simulink model "HvCoorn"  (R2022b)
settings: configuration reference "Icar05FusaMdlCfg" (kept outside this file)
undefined symbols (not defined in the file): BMSActSt_ACChrg, BMSActSt_DCChrg, BMSActSt_disconnect, BMSActSt_offline, BMSActSt_online, BMSActSt_undefined, BMSMainNegRlySt_Clsd_SC, BMSMainNegRlySt_Open_SC, BMSMainNegRlySt_StuckInClsd_SC, BMSMainNegRlySt_StuckInOpen_SC, BMSMainPosRlySt_Clsd_SC, BMSMainPosRlySt_Open_SC, BMSMainPosRlySt_StuckInClsd_SC, BMSPrecRlySt_StuckInOpen_SC, BMSReqSt_ACChrg, BMSReqSt_DCChrg, BMSReqSt_emergencyOffline, BMSReqSt_offline, BMSReqSt_online, Chrg_stCycleBookMod_SC, Chrg_stSingleBookMod_SC, CmpgMod_stInactv_SC, DCDCActSt_buck, DCDCActSt_connected, DCDCActSt_disconnected, DCDCReqSt_buck, DCDCReqSt_standby, EngStrtStop_RefuModDft_SC, EPBActSt_Appld_SC, GearLvr_stDrvGearD_SC, GearLvr_stDrvGearN_SC, GearLvr_stDrvGearP_SC, GearLvr_stDrvGearR_SC, hpp_bACChargeLinkIni_C, hpp_bACChargeLinkOKIni_C, hpp_bAcChgEnaIni_C, hpp_bAcChgPauseIni_C, hpp_bAcLinkTempErrIni_C, hpp_bBattWarmReqIni_C, hpp_bHvilHwErrIni_C, hpp_bHvilStOkIni_C, hpp_bHvRelayClsActIni_C, hpp_bHvRelayOpnActIni_C, hpp_bHvRelayStuckIni_C, hpp_bParked4ChDchgIni_C, hpp_bRemLvBatMntnReqIni_C, hpp_bStartUpReqIni_C, hpp_stHvilCanIni_C, hpp_stWarmTimeCfgRespIni_C, HvCoorn_bAuthEnaSwt_C, HvCoorn_bAuthFailSpdLimOvrd_C, HvCoorn_bAuthFailSpdLimOvrdVal_C, HvCoorn_bAuthStrt_C, HvCoorn_bBMSUnexpdDcnctFailEna_C, HvCoorn_bBuck2RdyBypDCDCEna_C, HvCoorn_bDCChrgFctCfg_C, HvCoorn_bDcChrgWkupEnaChrgLink_C, HvCoorn_bDCDcnct4ACEna_C, HvCoorn_bDCNotBuck2ShtdwnEna_C, HvCoorn_bDrvrLevNotRdyEna_C ... (+295)
libraries: ITKLib x213, simulink x61
(part 4 of 12)

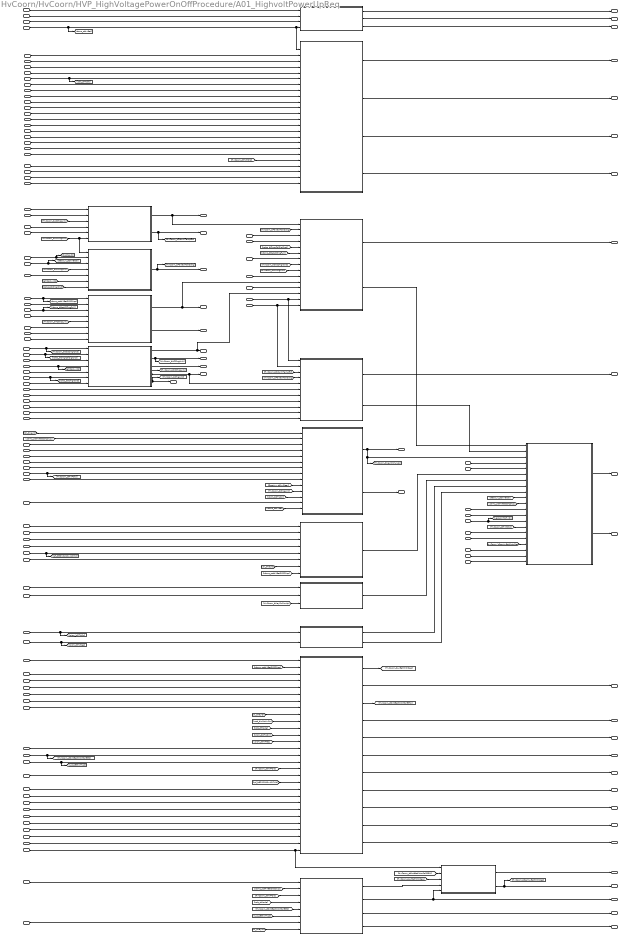
== system HvCoorn/HvCoorn/HVP_HighVoltagePowerOnOffProcedure/A01_HighvoltPowerUpReq ==
  HvCoorn_bHvReady : Inport
  BrkPedDev_bBrk : Inport  Port=2
  idi_bKeyOn : Inport  Port=3
  ian_tAcChrgrL1Temp : Inport  Port=4
  ian_tAcChrgrNTemp : Inport  Port=5
  icacu_stWarmTime : Inport  Port=6
  icbms_bBatACChrgFull : Inport  Port=7
  icbms_bStHvilSigErr : Inport  Port=8
  icbms_pctHVBatSOCDisp : Inport  Port=9
  icbms_stHvBat : Inport  Port=10
  icbms_stHvil : Inport  Port=11
  icbms_stMainNegRly : Inport  Port=12
  icbms_stMainPosRly : Inport  Port=13
  icbms_stPrecRly : Inport  Port=14
  icdc_bStHvilSigErr : Inport  Port=15
  icdc_stHvil : Inport  Port=16
  icdc_stMode : Inport  Port=17
  icfm_stMode : Inport  Port=18
  icobc_bChrgrCtrlSigCnct : Inport  Port=19
  icobc_bStAcHvilSigErr : Inport  Port=20
  icobc_pwrChrgMax : Inport  Port=21
  icobc_stHvil : Inport  Port=22
  HvCoorn_bObcChrgrCnct : Inport  Port=23
  icobc_stOBCMode : Inport  Port=24
  icobc_uChrgrCtrlSigVolt : Inport  Port=25
  icepb_stEpbSys : Inport  Port=26
  iczcu_stRmtChrgReq : Inport  Port=27
  Chrg_stBookChrgMod : Inport  Port=28
  ictel_stHvBatPrecdng : Inport  Port=29
  idi_bHvilInput : Inport  Port=30
  iud_bNoHVHWarmTiCfg : Inport  Port=31
  iud_bNoHVHConfig : Inport  Port=32
  iud_stOBCWakeUpOrigin : Inport  Port=33
  iud_stRemoteImmo : Inport  Port=34
  PwrLimBatt_pwrMaxHvesDChrg : Inport  Port=35
  Chrg_bACChrgCmpl : Inport  Port=36
  GearLvr_stDrvGear : Inport  Port=37
  VehSpd_vVeh : Inport  Port=38
  std_tExterTemp : Inport  Port=39
  HvCoorn_bHvilClsReqOld : Inport  Port=40
  tcj_bHvBatPrecdngFinish : Inport  Port=41
  inv_stHvBattWarmTime : Inport  Port=42
  icbms_stDcChrgrCnct : Inport  Port=43
  ian_tDcChrgrTemp1 : Inport  Port=44
  ian_tDcChrgrTemp2 : Inport  Port=45
  Chrg_bDCChrgCmpl : Inport  Port=46
  icbms_bBatDCChrgFull : Inport  Port=47
  icbms_uDcChgrCap : Inport  Port=48
  icbms_iDcChgrCap : Inport  Port=49
  icbms_bDcChrgCfg : Inport  Port=50
  icrm_stMode : Inport  Port=51
  VehCfg_bFrntMotByp : Inport  Port=52
  idi_bKeyStrt : Inport  Port=53
  icbms_bDcChrgWkup : Inport  Port=54
  Chrg_bChrgErrForever : Inport  Port=55
  icbms_bHvShutOffReq : Inport  Port=56
  iczcu_bHVPwrOffReq : Inport  Port=57
  icecc_bHVReq : Inport  Port=58
  HvCoorn_stHVPOld : Inport  Port=59
  icecc_bWPTCHvilFlt : Inport  Port=60
  icecc_bEASHvilFlt : Inport  Port=61
  icicm_bPwrOffReq : Inport  Port=62
  ved_bHvShtdwn : Inport  Port=63
  ipf_bBD1CAN0x41CVld : Inport  Port=64
  icicm_bOTAOn : Inport  Port=65
  icicm_stHVReq : Inport  Port=66
  icobc_bDchrgrCnct : Inport  Port=67
  ictcp_stRmtHvReq : Inport  Port=68
  iczcu_stCarMod : Inport  Port=69
  HvCoorn_bV2LActv : Inport  Port=70
  HvCoorn_bHvInitFail : Inport  Port=71
  HvCoorn_bHvOnFai : Inport  Port=72
  ved_bInhbHvOn : Inport  Port=73
  Chrg_bChrgStopBySOCLim : Inport  Port=74
  Chrg_bBookChrgCmpl : Inport  Port=75
  icobc_bVehCnct : Inport  Port=76
  icfm_bHvilFlt : Inport  Port=77
  icrm_bHvilFlt : Inport  Port=78
  icebs_pctLvBatSoh : Inport  Port=79
  icbms_tMaxBat : Inport  Port=80
  icbms_tMinBat : Inport  Port=81
  icebs_tLvBat : Inport  Port=82
  icebs_pctLvBatSoc : Inport  Port=83
  icebs_stSocPrcsn : Inport  Port=84
  icebs_uLvBat : Inport  Port=85
  icicm_stOTAPwrMngtReq : Inport  Port=86
  HvCoorn_ctSmtBatMntnFailEER : Inport  Port=87
  iud_bEEIniFnsd : Inport  Port=88
  HvCoorn_ctSmtBatMntnSucsEER : Inport  Port=89
  iclbms_stLvRemChrgReq : Inport  Port=90
  ipf_bLBMSCANVld : Inport  Port=91
  VehCfg_stLvBattTyp : Inport  Port=92
  icisg_bHvilFlt : Inport  Port=93
  idi_uPwrSply : Inport  Port=94
  ipf_bLIN9EBS0x34NodLostErr : Inport  Port=95
  HvCoorn_bSocWkupEER : Inport  Port=96
  HvCoorn_bTimerWkupReqEER : Inport  Port=97
  HvCoorn_stRemLvBatMntnFailRsnEER : Inport  Port=98
  icems_bFanAftRunActv : Inport  Port=99
  RngPrdn_volFuRmnByInstModEEW : Inport  Port=100
  ved_bInhbEngStrt : Inport  Port=101
  idi_bEBSLinWkup : Inport  Port=102
  idi_bTimerWkup : Inport  Port=103
  HvCoorn_pctHVBatSocEER : Inport  Port=104
  idi_noBMSSocCounter : Inport  Port=105
  DrvMod_bVehShowMod : Inport  Port=106
  icisg_uAct : Inport  Port=107
  icrm_uAct : Inport  Port=108
  icecc_uPTCAct : Inport  Port=109
  icecc_uEASAct : Inport  Port=110
  ved_bCellVoltUndLimSrus : Inport  Port=111
  B01_HvRelayClsAct : Subsystem  Description=高压继电器状态确认
  B02_HvilStCal : Subsystem  Description=互锁状态确认
  B03_ChgrPortOverTemp : Subsystem  Description=充电连接温度故障
  B04_ParkCheck : Subsystem  Description=停车检测
  B05_BattWarmReq : Subsystem
  B06_ChgrCnctStCal : Subsystem  Description=充电连接状态确认
  B07_AcChrgPwrUp : Subsystem  Description=AC充电上高压
  B08_DcChrgPwrUp : Subsystem  Description=DC充电上高压
  B09_KeyOnPwrUp : Subsystem  Description=KeyOn上高压
  B10_RemotePwrUp : Subsystem
  B11_ECCPwrUp : Subsystem  Description=热管理上高压
  B12_OTAPwrUp : Subsystem
  B13_GatherPwrUpReq : Subsystem  Description=高压上电请求
  B14_SmtLvBatMntn : Subsystem
  B15_LbmsMntn : Subsystem
  B16_LvBattTypSwt : Subsystem
  HvCoorn_bACChrgLink : Outport  VectorParamsAs1DForOutWhenUnconnected=off
  HvCoorn_bACChrgLinkOk : Outport  Port=2  VectorParamsAs1DForOutWhenUnconnected=off
  HvCoorn_stHvil : Outport  Port=3  VectorParamsAs1DForOutWhenUnconnected=off
  HvCoorn_bHvilHwStOk : Outport  Port=4  VectorParamsAs1DForOutWhenUnconnected=off
  HvCoorn_bHvilStOk : Outport  Port=5  VectorParamsAs1DForOutWhenUnconnected=off
  HvCoorn_bACChrgPause : Outport  Port=6  VectorParamsAs1DForOutWhenUnconnected=off
  HvCoorn_bHvRlyClsAct : Outport  Port=7  VectorParamsAs1DForOutWhenUnconnected=off
  HvCoorn_bHvRlyOpenAct : Outport  Port=8  VectorParamsAs1DForOutWhenUnconnected=off
  HvCoorn_bHvRlyStuck : Outport  Port=9  VectorParamsAs1DForOutWhenUnconnected=off
  HvCoorn_bACLinkTempErr : Outport  Port=10  VectorParamsAs1DForOutWhenUnconnected=off
  HvCoorn_bParked4ChDchg : Outport  Port=11  VectorParamsAs1DForOutWhenUnconnected=off
  HvCoorn_bBattWarmReq : Outport  Port=12  VectorParamsAs1DForOutWhenUnconnected=off
  HvCoorn_stWarmTimeCfgResp : Outport  Port=13  VectorParamsAs1DForOutWhenUnconnected=off
  HvCoorn_bACChrgEna : Outport  Port=14  VectorParamsAs1DForOutWhenUnconnected=off
  HvCoorn_bRemLvBatMntnReq : Outport  Port=15  VectorParamsAs1DForOutWhenUnconnected=off
  HvCoorn_bDCChrgLink : Outport  Port=16  VectorParamsAs1DForOutWhenUnconnected=off
  HvCoorn_bChrgLink : Outport  Port=17  VectorParamsAs1DForOutWhenUnconnected=off
  HvCoorn_bDCLinkTempErr : Outport  Port=18  VectorParamsAs1DForOutWhenUnconnected=off
  HvCoorn_bDCChrgEna : Outport  Port=19  VectorParamsAs1DForOutWhenUnconnected=off
  HvCoorn_stStartUpReq : Outport  Port=20  VectorParamsAs1DForOutWhenUnconnected=off
  HvCoorn_bCtrlrHvilErr : Outport  Port=21  VectorParamsAs1DForOutWhenUnconnected=off
  HvCoorn_bKeyOnPwrUp : Outport  Port=22  VectorParamsAs1DForOutWhenUnconnected=off
  HvCoorn_bSocWkup : Outport  Port=23  VectorParamsAs1DForOutWhenUnconnected=off
  HvCoorn_ctSmtBatMntnFailEEW : Outport  Port=24  VectorParamsAs1DForOutWhenUnconnected=off
  HvCoorn_stRemLvBatMntnFailRsn : Outport  Port=25  VectorParamsAs1DForOutWhenUnconnected=off
  HvCoorn_ctSmtBatMntnSucsEEW : Outport  Port=26  VectorParamsAs1DForOutWhenUnconnected=off
  HvCoorn_bTimerWkupReq : Outport  Port=27  VectorParamsAs1DForOutWhenUnconnected=off
  HvCoorn_bLbmsLvBatMntnReq : Outport  Port=28  VectorParamsAs1DForOutWhenUnconnected=off
  HvCoorn_pctLbmsSocMntnThd : Outport  Port=29  VectorParamsAs1DForOutWhenUnconnected=off
  HvCoorn_bLbmsSocWkup : Outport  Port=30  VectorParamsAs1DForOutWhenUnconnected=off
  HvCoorn_bVehNetWkupEna : Outport  Port=31  VectorParamsAs1DForOutWhenUnconnected=off
  HvCoorn_bSocWkupEEW : Outport  Port=32  VectorParamsAs1DForOutWhenUnconnected=off
  HvCoorn_bTimerWkupReqEEW : Outport  Port=33  VectorParamsAs1DForOutWhenUnconnected=off
  HvCoorn_stRemLvBatMntnFailRsnEEW : Outport  Port=34  VectorParamsAs1DForOutWhenUnconnected=off
  HvCoorn_pctHVBatSocEEW : Outport  Port=35  VectorParamsAs1DForOutWhenUnconnected=off
  HvCoorn_bShowModSocLo : Outport  Port=36  VectorParamsAs1DForOutWhenUnconnected=off
  HvCoorn_bStartUpReq : Outport  Port=37  VectorParamsAs1DForOutWhenUnconnected=off
  wires:
  B06_ChgrCnctStCal/2(HvCoorn_bACChrgLink) -> [HvCoorn_bACChrgLink], HvCoorn_bACChrgLink/1
  icdc_bStHvilSigErr/1 -> B02_HvilStCal/3(icdc_bStHvilSigErr)
  icobc_bStAcHvilSigErr/1 -> B02_HvilStCal/4(icobc_bStAcHvilSigErr)
  icbms_bStHvilSigErr/1 -> B02_HvilStCal/2(icbms_bStHvilSigErr)
  icdc_stMode/1 -> [icdc_stMode], B02_HvilStCal/6(icdc_stMode)
  icobc_stOBCMode/1 -> B02_HvilStCal/7(icobc_stOBCMode)
  idi_bHvilInput/1 -> B02_HvilStCal/8(idi_bHvilInput)
  icbms_stHvil/1 -> B02_HvilStCal/9(icbms_stHvil)
  icdc_stHvil/1 -> B02_HvilStCal/10(icdc_stHvil)
  icobc_stHvil/1 -> B02_HvilStCal/11(icobc_stHvil)
  B02_HvilStCal/3(HvCoorn_stHvil) -> HvCoorn_stHvil/1
  B02_HvilStCal/2(HvCoorn_bHvilHwStOk) -> HvCoorn_bHvilHwStOk/1
  B02_HvilStCal/1(HvCoorn_bHvilStOk) -> HvCoorn_bHvilStOk/1
  HvCoorn_bObcChrgrCnct/1 -> B06_ChgrCnctStCal/1(HvCoorn_bObcChrgrCnct), [HvCoorn_bObcChrgrCnct]
  icobc_bChrgrCtrlSigCnct/1 -> B06_ChgrCnctStCal/2(icobc_bChrgrCtrlSigCnct), [icobc_bChrgrCtrlSigCnct]
  VehSpd_vVeh/1 -> [VehSpd_vVeh], B06_ChgrCnctStCal/4(VehSpd_vVeh)
  icobc_uChrgrCtrlSigVolt/1 -> B06_ChgrCnctStCal/3(icobc_uChrgrCtrlSigVolt)
  B06_ChgrCnctStCal/3(HvCoorn_bACChrgPause) -> HvCoorn_bACChrgPause/1
  icfm_stMode/1 -> B02_HvilStCal/5(icfm_stMode)
  icbms_stHvBat/1 -> [icbms_stHvBat], B02_HvilStCal/1(icbms_stHvBat), B01_HvRelayClsAct/4(icbms_stHvBat)
  icbms_stMainPosRly/1 -> B01_HvRelayClsAct/1(icbms_stMainPosRly)
  icbms_stPrecRly/1 -> B01_HvRelayClsAct/2(icbms_stPrecRly)
  icbms_stMainNegRly/1 -> B01_HvRelayClsAct/3(icbms_stMainNegRly)
  B01_HvRelayClsAct/1(HvCoorn_bHvRlyClsAct) -> HvCoorn_bHvRlyClsAct/1
  B01_HvRelayClsAct/2(HvCoorn_bHvRlyOpenAct) -> HvCoorn_bHvRlyOpenAct/1
  B01_HvRelayClsAct/3(HvCoorn_bHvRlyStuck) -> HvCoorn_bHvRlyStuck/1
  ian_tAcChrgrL1Temp/1 -> B03_ChgrPortOverTemp/1(ian_tAcChrgrL1Temp)
  ian_tAcChrgrNTemp/1 -> B03_ChgrPortOverTemp/2(ian_tAcChrgrNTemp)
  [HvCoorn_bACChrgLink] -> B03_ChgrPortOverTemp/3(HvCoorn_bACChrgLink)
  [HvCoorn_bACChrgLink] -> B04_ParkCheck/4(HvCoorn_bACChrgLink)
  icepb_stEpbSys/1 -> B04_ParkCheck/5(icepb_stEpbSys)
  GearLvr_stDrvGear/1 -> B04_ParkCheck/3(GearLvr_stDrvGear), [GearLvr_stDrvGear]
  idi_bKeyOn/1 -> B04_ParkCheck/2(idi_bKeyOn), [idi_bKeyOn]
  Chrg_stBookChrgMod/1 -> B07_AcChrgPwrUp/7(Chrg_stBookChrgMod)
  B05_BattWarmReq/1(HvCoorn_bBattWarmReq) -> HvCoorn_bBattWarmReq/1, B07_AcChrgPwrUp/11(HvCoorn_bBattWarmReq)
  std_tExterTemp/1 -> B05_BattWarmReq/2(std_tExterTemp)
  [HvCoorn_bACChrgLink] -> B05_BattWarmReq/5(HvCoorn_bACChrgLink)
  icbms_bBatACChrgFull/1 -> [icbms_bBatACChrgFull], B05_BattWarmReq/3(icbms_bBatACChrgFull)
  B05_BattWarmReq/2(HvCoorn_stWarmTimeCfgResp) -> HvCoorn_stWarmTimeCfgResp/1
  icacu_stWarmTime/1 -> B05_BattWarmReq/4(icacu_stWarmTime)
  icbms_pctHVBatSOCDisp/1 -> B05_BattWarmReq/1(icbms_pctHVBatSOCDisp), [icbms_pctHVBatSOCDisp]
  B07_AcChrgPwrUp/1(HvCoorn_bACChrgEna) -> HvCoorn_bACChrgEna/1
  B03_ChgrPortOverTemp/1(HvCoorn_bACLinkTempErr) -> HvCoorn_bACLinkTempErr/1, B07_AcChrgPwrUp/1(HvCoorn_bACLinkTempErr)
  HvCoorn_bHvilClsReqOld/1 -> B02_HvilStCal/12(HvCoorn_bHvilClsReq)
  iud_bNoHVHConfig/1 -> B05_BattWarmReq/6(iud_bNoHVHConfig)
  iud_bNoHVHWarmTiCfg/1 -> B05_BattWarmReq/7(iud_bNoHVHWarmTiCfg)
  inv_stHvBattWarmTime/1 -> B05_BattWarmReq/8(inv_stHvBattWarmTime)
  PwrLimBatt_pwrMaxHvesDChrg/1 -> B09_KeyOnPwrUp/3(PwrLimBatt_pwrMaxHvesDChrg)
  [icbms_pctHVBatSOCDisp] -> B09_KeyOnPwrUp/2(icbms_pctHVBatSOCDisp)
  iud_stRemoteImmo/1 -> B10_RemotePwrUp/4(iud_stRemoteImmo)
  iczcu_stRmtChrgReq/1 -> B10_RemotePwrUp/3(iczcu_stRmtChrgReq)
  tcj_bHvBatPrecdngFinish/1 -> B10_RemotePwrUp/2(tcj_bHvBatPrecdngFinish)
  ictel_stHvBatPrecdng/1 -> B10_RemotePwrUp/1(ictel_stHvBatPrecdng)
  B10_RemotePwrUp/1(HvCoorn_bRemPwrUp) -> B13_GatherPwrUpReq/6(HvCoorn_bRemPwrUp)
  B09_KeyOnPwrUp/1(HvCoorn_bKeyOnPwrUp) -> [HvCoorn_bKeyOnPwrUp], B13_GatherPwrUpReq/3(HvCoorn_bKeyOnPwrUp), HvCoorn_bKeyOnPwrUp/1
  B07_AcChrgPwrUp/2(HvCoorn_bACChrgPwrUp) -> B13_GatherPwrUpReq/1(HvCoorn_bACChrgPwrUp)
  [idi_bKeyOn] -> B09_KeyOnPwrUp/1(idi_bKeyOn)
  icobc_pwrChrgMax/1 -> B07_AcChrgPwrUp/10(icobc_pwrChrgMax)
  [HvCoorn_bObcChrgrCnct] -> B07_AcChrgPwrUp/8(HvCoorn_bObcChrgrCnct)
  [icbms_bBatACChrgFull] -> B07_AcChrgPwrUp/6(icbms_bBatACChrgFull)
  [icobc_bChrgrCtrlSigCnct] -> B07_AcChrgPwrUp/5(icobc_bChrgrCtrlSigCnct)
  iud_stOBCWakeUpOrigin/1 -> B07_AcChrgPwrUp/4(iud_stOBCWakeUpOrigin)
  Chrg_bACChrgCmpl/1 -> B07_AcChrgPwrUp/3(Chrg_bACChrgCmpl)
  [HvCoorn_bACChrgLink] -> B07_AcChrgPwrUp/9(HvCoorn_bACChrgLink)
  B06_ChgrCnctStCal/1(HvCoorn_bACChrgLinkOk) -> HvCoorn_bACChrgLinkOk/1, B07_AcChrgPwrUp/13(HvCoorn_bACChrgLinkOk)
  icbms_stDcChrgrCnct/1 -> B06_ChgrCnctStCal/5(icbms_stDcChrgrCnct)
  B06_ChgrCnctStCal/4(HvCoorn_bDCChrgLink) -> [HvCoorn_bDCChrgLink], HvCoorn_bDCChrgLink/1, B08_DcChrgPwrUp/5(HvCoorn_bDCChrgLink)
  B06_ChgrCnctStCal/5(HvCoorn_bChrgLink) -> [HvCoorn_bChrgLink], HvCoorn_bChrgLink/1
  B08_DcChrgPwrUp/2(HvCoorn_bDCChrgPwrUp) -> B13_GatherPwrUpReq/2(HvCoorn_bDCChrgPwrUp)
  [HvCoorn_bDCChrgLink] -> B04_ParkCheck/1(HvCoorn_bDCChrgLink), B03_ChgrPortOverTemp/6(HvCoorn_bDCChargeLink)
  ian_tDcChrgrTemp1/1 -> B03_ChgrPortOverTemp/4(ian_tDcChrgrTemp1)
  ian_tDcChrgrTemp2/1 -> B03_ChgrPortOverTemp/5(ian_tDcChrgrTemp2)
  B03_ChgrPortOverTemp/2(HvCoorn_bDCLinkTempErr) -> [HvCoorn_bDcLinkTempErr], HvCoorn_bDCLinkTempErr/1
  [HvCoorn_bDcLinkTempErr] -> B08_DcChrgPwrUp/3(HvCoorn_bDcLinkTempErr)
  [HvCoorn_bParked4ChDchg] -> B08_DcChrgPwrUp/4(HvCoorn_bParked4ChDchg)
  B04_ParkCheck/1(HvCoorn_bParked4ChDchg) -> HvCoorn_bParked4ChDchg/1, [HvCoorn_bParked4ChDchg]
  icbms_bDcChrgCfg/1 -> B08_DcChrgPwrUp/6(icbms_bDcChrgCfg)
  Chrg_bDCChrgCmpl/1 -> B08_DcChrgPwrUp/7(Chrg_bDCChrgCmpl)
  icbms_bBatDCChrgFull/1 -> B08_DcChrgPwrUp/8(icbms_bBatDCChrgFull)
  icbms_uDcChgrCap/1 -> B08_DcChrgPwrUp/9(icbms_uDcChgrCap)
  icbms_iDcChgrCap/1 -> B08_DcChrgPwrUp/10(icbms_iDcChgrCap)
  B08_DcChrgPwrUp/1(HvCoorn_bDCChrgEna) -> HvCoorn_bDCChrgEna/1
  [HvCoorn_bParked4ChDchg] -> B07_AcChrgPwrUp/2(HvCoorn_bParked4ChDchg)
  icrm_stMode/1 -> B02_HvilStCal/13(icrm_stMode)
  VehCfg_bFrntMotByp/1 -> B02_HvilStCal/14(VehCfg_bFrntMotByp)
  idi_bKeyStrt/1 -> B09_KeyOnPwrUp/4(idi_bKeyStrt)
  icbms_bDcChrgWkup/1 -> B08_DcChrgPwrUp/11(icbms_bDcChrgWkup)
  HvCoorn_bHvReady/1 -> B09_KeyOnPwrUp/5(HvCoorn_bHvReady)
  BrkPedDev_bBrk/1 -> B09_KeyOnPwrUp/6(BrkPedDev_bBrk)
  [VehSpd_vVeh] -> B04_ParkCheck/6(VehSpd_vVeh)
  Chrg_bChrgErrForever/1 -> B08_DcChrgPwrUp/2(Chrg_bChrgErrForever), B07_AcChrgPwrUp/15(Chrg_bChrgErrForever)
  icbms_bHvShutOffReq/1 -> B13_GatherPwrUpReq/5(icbms_bHvShutOffReq)
  iczcu_bHVPwrOffReq/1 -> B09_KeyOnPwrUp/7(iczcu_bHVPwrOffReq)
  icecc_bHVReq/1 -> B11_ECCPwrUp/1(icecc_bHVReq)
  B11_ECCPwrUp/1(HvCoorn_bECCPwrUp) -> B13_GatherPwrUpReq/7(HvCoorn_bECCPwrUp)
  B13_GatherPwrUpReq/1(HvCoorn_bStartUpReq) -> HvCoorn_bStartUpReq/1
  HvCoorn_stHVPOld/1 -> [HvCoorn_stHVPOld], B09_KeyOnPwrUp/8(HvCoorn_stHVPOld)
  icecc_bWPTCHvilFlt/1 -> B02_HvilStCal/15(icecc_bWPTCHvilFlt)
  icecc_bEASHvilFlt/1 -> B02_HvilStCal/16(icecc_bEASHvilFlt)
  icicm_bPwrOffReq/1 -> B09_KeyOnPwrUp/9(icicm_bPwrOffReq)
  ved_bHvShtdwn/1 -> B13_GatherPwrUpReq/4(ved_bHvShtdwn)
  ipf_bBD1CAN0x41CVld/1 -> [ipf_bBD1CAN0x41CVld], B10_RemotePwrUp/5(ipf_bBD1CAN0x41CVld)
  icicm_bOTAOn/1 -> [icicm_bOTAOn], B12_OTAPwrUp/1(icicm_bOTAOn)
  icicm_stHVReq/1 -> [icicm_stHVReq], B12_OTAPwrUp/2(icicm_stHVReq)
  B12_OTAPwrUp/1(HvCoorn_bOTAPwrUp) -> B13_GatherPwrUpReq/8(HvCoorn_bOTAPwrUp)
  B12_OTAPwrUp/2(HvCoorn_bOTAHvOffReq) -> B13_GatherPwrUpReq/9(HvCoorn_bOTAHvOffReq)
  icobc_bDchrgrCnct/1 -> [icobc_bDchrgrCnct], B06_ChgrCnctStCal/6(icobc_bDchrgrCnct)
  B13_GatherPwrUpReq/2(HvCoorn_stStartUpReq) -> HvCoorn_stStartUpReq/1
  ictcp_stRmtHvReq/1 -> B10_RemotePwrUp/6(ictcp_stRmtHvReq)
  [icobc_bDchrgrCnct] -> B04_ParkCheck/7(icobc_bDchrgrCnct)
  [icbms_pctHVBatSOCDisp] -> B13_GatherPwrUpReq/11(icbms_pctHVBatSOCDisp)
  [GearLvr_stDrvGear] -> B13_GatherPwrUpReq/10(GearLvr_stDrvGear)
  iczcu_stCarMod/1 -> B13_GatherPwrUpReq/12(iczcu_stCarMod)
  HvCoorn_bV2LActv/1 -> B13_GatherPwrUpReq/13(HvCoorn_bV2LActv)
  [GearLvr_stDrvGear] -> B09_KeyOnPwrUp/10(GearLvr_stDrvGear)
  [idi_bKeyOn] -> B10_RemotePwrUp/7(idi_bKeyOn)
  [HvCoorn_bChrgLink] -> B09_KeyOnPwrUp/11(HvCoorn_bChrgLink)
  [HvCoorn_stHVPOld] -> B13_GatherPwrUpReq/15(HvCoorn_stHVPOld)
  ved_bInhbHvOn/1 -> [ved_bInhbHvOn], B13_GatherPwrUpReq/14(ved_bInhbHvOn)
  HvCoorn_bHvOnFai/1 -> B13_GatherPwrUpReq/16(HvCoorn_bHvOnFai)
  HvCoorn_bHvInitFail/1 -> B13_GatherPwrUpReq/17(HvCoorn_bHvInitFail)
  Chrg_bChrgStopBySOCLim/1 -> B08_DcChrgPwrUp/1(Chrg_bChrgStopBySOCLim), B07_AcChrgPwrUp/14(Chrg_bChrgStopBySOCLim)
  Chrg_bBookChrgCmpl/1 -> B07_AcChrgPwrUp/12(Chrg_bBookChrgCmpl)
  icobc_bVehCnct/1 -> B06_ChgrCnctStCal/7(icobc_bVehCnct)
  B02_HvilStCal/4(HvCoorn_bCtrlrHvilErr) -> HvCoorn_bCtrlrHvilErr/1
  icfm_bHvilFlt/1 -> B02_HvilStCal/17(icfm_bHvilFlt)
  icrm_bHvilFlt/1 -> B02_HvilStCal/18(icrm_bHvilFlt)
  B14_SmtLvBatMntn/1(HvCoorn_bLvBatMntnReq) -> [HvCoorn_bLvBatMntnReq]
  HvCoorn_ctSmtBatMntnFailEER/1 -> B14_SmtLvBatMntn/15(HvCoorn_ctSmtBatMntnFailEER), [HvCoorn_ctSmtBatMntnFailEER]
  iud_bEEIniFnsd/1 -> B14_SmtLvBatMntn/16(iud_bEEIniFnsd), [iud_bEEIniFnsd]
  B14_SmtLvBatMntn/2(HvCoorn_bSocWkup) -> HvCoorn_bSocWkup/1
  icbms_tMinBat/1 -> B14_SmtLvBatMntn/4(icbms_tMinBat)
  icebs_stSocPrcsn/1 -> B14_SmtLvBatMntn/7(icebs_stSocPrcsn)
  [icicm_stHVReq] -> B14_SmtLvBatMntn/13(icicm_stHVReq)
  icebs_pctLvBatSoh/1 -> B14_SmtLvBatMntn/1(icebs_pctLvBatSoh)
  [icdc_stMode] -> B14_SmtLvBatMntn/11(icdc_stMode)
  [icicm_bOTAOn] -> B14_SmtLvBatMntn/12(icicm_bOTAOn)
  [icbms_pctHVBatSOCDisp] -> B14_SmtLvBatMntn/2(icbms_pctHVBatSOCDisp)
  icicm_stOTAPwrMngtReq/1 -> B14_SmtLvBatMntn/14(icicm_stOTAPwrMngtReq)
  icebs_pctLvBatSoc/1 -> B14_SmtLvBatMntn/6(icebs_pctLvBatSoc)
  [idi_bKeyOn] -> B14_SmtLvBatMntn/9(idi_bKeyOn)
  icbms_tMaxBat/1 -> B14_SmtLvBatMntn/3(icbms_tMaxBat)
  icebs_uLvBat/1 -> B14_SmtLvBatMntn/8(icebs_uLvBat)
  icebs_tLvBat/1 -> B14_SmtLvBatMntn/5(icebs_tLvBat)
  [HvCoorn_stHVPOld] -> B14_SmtLvBatMntn/17(HvCoorn_stHVPOld)
  HvCoorn_ctSmtBatMntnSucsEER/1 -> B14_SmtLvBatMntn/18(HvCoorn_ctSmtBatMntnSucsEER)
  B14_SmtLvBatMntn/4(HvCoorn_stRemLvBatMntnFailRsn) -> HvCoorn_stRemLvBatMntnFailRsn/1
  B14_SmtLvBatMntn/5(HvCoorn_bTimerWkupReq) -> HvCoorn_bTimerWkupReq/1
  [icbms_pctHVBatSOCDisp] -> B15_LbmsMntn/2(icbms_pctHVBatSOCDisp)
  iclbms_stLvRemChrgReq/1 -> B15_LbmsMntn/1(iclbms_stLvRemChrgReq)
  [HvCoorn_stHVPOld] -> B15_LbmsMntn/3(HvCoorn_stHVPOld)
  [icdc_stMode] -> B15_LbmsMntn/4(icdc_stMode)
  [iud_bEEIniFnsd] -> B15_LbmsMntn/6(iud_bEEIniFnsd)
  ipf_bLBMSCANVld/1 -> B15_LbmsMntn/7(ipf_bLBMSCANVld)
  [HvCoorn_ctSmtBatMntnFailEER] -> B15_LbmsMntn/5(HvCoorn_ctSmtBatMntnFailEER)
  B15_LbmsMntn/3(HvCoorn_pctLbmsSocMntnThd) -> HvCoorn_pctLbmsSocMntnThd/1
  B15_LbmsMntn/4(HvCoorn_bLbmsSocWkup) -> HvCoorn_bLbmsSocWkup/1
  B15_LbmsMntn/2(HvCoorn_bLbmsLvBatMntnReq) -> B16_LvBattTypSwt/5(HvCoorn_bLbmsLvBatMntnReq), HvCoorn_bLbmsLvBatMntnReq/1
  VehCfg_stLvBattTyp/1 -> B14_SmtLvBatMntn/29(VehCfg_stLvBattTyp), B16_LvBattTypSwt/1(VehCfg_stLvBattTyp)
  B15_LbmsMntn/1(HvCoorn_ctLbmsMntnFailEEW) -> B16_LvBattTypSwt/4(HvCoorn_ctLbmsMntnFailEEW)
  B14_SmtLvBatMntn/6(HvCoorn_ctSmtBatMntnSucsEEW) -> HvCoorn_ctSmtBatMntnSucsEEW/1
  B14_SmtLvBatMntn/3(HvCoorn_ctSmtBatMntnFailEEW) -> [HvCoorn_ctSmtBatMntnFailEEW]
  B16_LvBattTypSwt/1(HvCoorn_ctSmtBatMntnFailEEW) -> HvCoorn_ctSmtBatMntnFailEEW/1
  [HvCoorn_ctSmtBatMntnFailEEW] -> B16_LvBattTypSwt/2(HvCoorn_ctSmtBatMntnFailEEW1)
  [HvCoorn_bRemLvBatMntnReq] -> B13_GatherPwrUpReq/18(HvCoorn_bRemLvBatMntnReq)
  [HvCoorn_bLvBatMntnReq] -> B16_LvBattTypSwt/3(HvCoorn_bLvBatMntnReq)
  B16_LvBattTypSwt/2(HvCoorn_bRemLvBatMntnReq) -> [HvCoorn_bRemLvBatMntnReq], HvCoorn_bRemLvBatMntnReq/1
  icisg_bHvilFlt/1 -> B02_HvilStCal/19(icisg_bHvilFlt)
  [ipf_bBD1CAN0x41CVld] -> B14_SmtLvBatMntn/19(ipf_bBD1CAN0x41CVld)
  idi_uPwrSply/1 -> B14_SmtLvBatMntn/20(idi_uPwrSply)
  [ved_bInhbHvOn] -> B14_SmtLvBatMntn/10(ved_bInhbHvOn)
  B14_SmtLvBatMntn/7(HvCoorn_bVehNetWkupEna) -> HvCoorn_bVehNetWkupEna/1
  ipf_bLIN9EBS0x34NodLostErr/1 -> B14_SmtLvBatMntn/21(ipf_bLIN9EBS0x34NodLostErr)
  [icicm_bOTAOn] -> B09_KeyOnPwrUp/12(icicm_bOTAOn)
  HvCoorn_bSocWkupEER/1 -> B14_SmtLvBatMntn/22(HvCoorn_bSocWkupEER)
  HvCoorn_bTimerWkupReqEER/1 -> B14_SmtLvBatMntn/23(HvCoorn_bTimerWkupReqEER)
  B14_SmtLvBatMntn/8(HvCoorn_bSocWkupEEW) -> HvCoorn_bSocWkupEEW/1
  B14_SmtLvBatMntn/9(HvCoorn_bTimerWkupReqEEW) -> HvCoorn_bTimerWkupReqEEW/1
  HvCoorn_stRemLvBatMntnFailRsnEER/1 -> B14_SmtLvBatMntn/24(HvCoorn_stRemLvBatMntnFailRsnEER)
  B14_SmtLvBatMntn/10(HvCoorn_stRemLvBatMntnFailRsnEEW) -> HvCoorn_stRemLvBatMntnFailRsnEEW/1
  [idi_bKeyOn] -> B15_LbmsMntn/8(idi_bKeyOn)
  [HvCoorn_bKeyOnPwrUp] -> B11_ECCPwrUp/3(HvCoorn_bKeyOnPwrUp)
  icems_bFanAftRunActv/1 -> B11_ECCPwrUp/2(icems_bFanAftRunActv)
  RngPrdn_volFuRmnByInstModEEW/1 -> B13_GatherPwrUpReq/19(RngPrdn_volFuRmnByInstModEEW)
  ved_bInhbEngStrt/1 -> B13_GatherPwrUpReq/20(ved_bInhbEngStrt)
  idi_bEBSLinWkup/1 -> B14_SmtLvBatMntn/25(idi_bEBSLinWkup)
  idi_bTimerWkup/1 -> B14_SmtLvBatMntn/26(idi_bTimerWkup)
  HvCoorn_pctHVBatSocEER/1 -> B14_SmtLvBatMntn/27(HvCoorn_pctHVBatSocEER)
  idi_noBMSSocCounter/1 -> B14_SmtLvBatMntn/28(idi_noBMSSocCounter)
  B14_SmtLvBatMntn/11(HvCoorn_pctHVBatSocEEW) -> HvCoorn_pctHVBatSocEEW/1
  DrvMod_bVehShowMod/1 -> B09_KeyOnPwrUp/13(DrvMod_bVehShowMod)
  [icbms_stHvBat] -> B09_KeyOnPwrUp/14(icbms_stHvBat)
  B09_KeyOnPwrUp/2(HvCoorn_bShowModSocLo) -> HvCoorn_bShowModSocLo/1
  [HvCoorn_stHVPOld] -> B02_HvilStCal/20(HvCoorn_stHVPOld)
  icisg_uAct/1 -> B02_HvilStCal/21(icisg_uAct)
  icrm_uAct/1 -> B02_HvilStCal/22(icrm_uAct)
  icecc_uPTCAct/1 -> B02_HvilStCal/23(icecc_uPTCAct)
  icecc_uEASAct/1 -> B02_HvilStCal/24(icecc_uEASAct)
  [icbms_pctHVBatSOCDisp] -> B10_RemotePwrUp/8(icbms_pctHVBatSOCDisp)
  ved_bCellVoltUndLimSrus/1 -> B13_GatherPwrUpReq/21(ved_bCellVoltUndLimSrus)

== system HvCoorn/HvCoorn/HVP_HighVoltagePowerOnOffProcedure/A02_Init2StupCal ==
  note: This subsystem calculates the timer of high voltage power on or off status and the transmission flag from initial status to start up status.
  note: Documentation
  HvCoorn_bStartUpReq : Inport
  HvCoorn_bHvOnFail : Inport  Port=2
  HvCoorn_bDischargeErrOld : Inport  Port=3
  HvCoorn_bHvInitFail : Inport  Port=4
  HvCoorn_stHVPOld : Inport  Port=5
  HvCoorn_bHvRlyOpenAct : Inport  Port=6
  AND : Logic  Inputs=3  OutDataTypeStr=boolean
  Copyright : simulink/Model-Wide Utilities/Model Info  Frame=on  DisplayStringWithTags=|  HorizontalTextAlignment=Left  LeftAlignmentValue=0.02
      | © ITK Engineering Technology (Wu Xi) Co., Ltd. (ITKC)
      | 
      | Model Version: %<ModelVersion>
      | Date: %<LastModificationDate>
  DataTypeConversion : DataTypeConversion  OutDataTypeStr=single  SaturateOnIntegerOverflow=off  RndMeth=Floor
  InlineDescription : ITKLib/Special/InlineDescription  Tag=HideFromReport  Description=初始化跳转至上高压  ShowInLibBrowser=0  RefreshPar=0
      settings: SourceProductName=ITKC_Lib
  Logical Operator : Logic  Inputs=4  AllPortsSameDT=off  OutDataTypeStr=boolean
  Logical Operator1 : Logic  Operator=NOT  Inputs=1  AllPortsSameDT=off  OutDataTypeStr=boolean
  Logical Operator3 : Logic  Operator=NOT  Inputs=1  AllPortsSameDT=off  OutDataTypeStr=boolean
  Logical Operator4 : Logic  Operator=NOT  Inputs=1  AllPortsSameDT=off  OutDataTypeStr=boolean
  MinMax : MinMax  Inputs=2  SaturateOnIntegerOverflow=on
  OR : Logic  Operator=OR  OutDataTypeStr=boolean
  OR1 : Logic  Operator=OR  OutDataTypeStr=boolean
  Relational Operator : RelationalOperator  Operator=>  OutDataTypeStr=boolean  InputSameDT=off
  Relational Operator2 : RelationalOperator  Operator=~=  OutDataTypeStr=boolean  InputSameDT=off
  Sum1 : Sum  OutDataTypeStr=uint32  SaturateOnIntegerOverflow=on
  Switch : Switch  Criteria=u2 ~= 0  SaturateOnIntegerOverflow=off  InputSameDT=off
  TaskTime_s2 : Constant  Value=TaskTime_10ms
      settings: AttributesFormatString=[0.01]
  Unit Delay1 : UnitDelay  SampleTime=-1  HasFrameUpgradeWarning=on
      settings: AttributesFormatString=<initial=%<X0>>
  Unit Delay2 : UnitDelay  SampleTime=-1  HasFrameUpgradeWarning=on
      settings: AttributesFormatString=<initial=%<X0>>
  Unit detailed design : simulink/Model-Wide Utilities/DocBlock  Tag=HideFromReport  DocumentType=Text
      content=|
      | SMiVCU-3278 - 状态持续时间
      | 当前时刻<高压系统状态>与上一时刻一致，则开始进行计时累加得到[状态持续时间]，当前时刻<高压系统状态>与上一时刻不一致，则计时清零。
      |
      | SMiVCU-3279 - 初始化至上高压标志位
      | 若以下条件同时满足，则激活[初始化至上高压标志位]：
      | 1.[状态持续时间]大于一定值（HvCoorn_tiWaitIgnOn_C，0.05s）；
      | 2.[上高压需求标志位]为1；
      | 3.[上高压失败标志位]为0；
      | 4.[放电失败标志位]为0；
      | 5.[高压初始化失败标志位]为0；
  product : Product  Inputs=**  RndMeth=Zero  SaturateOnIntegerOverflow=on
  sup_tiWaitIgnOn_C : Constant  Description=[0]  Value=HvCoorn_tiWaitIgnOn_C
      settings: AttributesFormatString=%<Description>
  sup_tiWaitIgnOn_C1 : Constant  Description=[1]  Value=HvCoorn_bInitErrChkByp_C
      settings: AttributesFormatString=%<Description>
  sup_tiWaitIgnOn_C2 : Constant  Description=[1]  Value=HvCoorn_bInitRlyOpenChkByp_C
      settings: AttributesFormatString=%<Description>
  uint1 : Constant  OutDataTypeStr=uint32
      settings: AttributesFormatString=%<OutDataTypeStr>
  uint2 : Constant  Value=65535  OutDataTypeStr=uint32
      settings: AttributesFormatString=%<OutDataTypeStr>
  uint32 : Constant  Value=0  OutDataTypeStr=uint32
      settings: AttributesFormatString=%<OutDataTypeStr>
  HvCoorn_tiHVPStTimer : Outport  VectorParamsAs1DForOutWhenUnconnected=off
  HvCoorn_bInit2StrtUp : Outport  Port=2  VectorParamsAs1DForOutWhenUnconnected=off
  wires:
  HvCoorn_bStartUpReq/1 -> Logical Operator/2
  Logical Operator/1 -> HvCoorn_bInit2StrtUp/1  "HvCoorn_bInit2StrtUp"
  sup_tiWaitIgnOn_C/1 -> Relational Operator/2
  Relational Operator/1 -> Logical Operator/1
  HvCoorn_bHvOnFail/1 -> Logical Operator3/1
  Logical Operator3/1 -> AND/1
  HvCoorn_bDischargeErrOld/1 -> Logical Operator4/1
  Logical Operator4/1 -> AND/2
  HvCoorn_bHvInitFail/1 -> Logical Operator1/1
  Logical Operator1/1 -> AND/3
  TaskTime_s2/1 -> product/2
  HvCoorn_stHVPOld/1 -> Unit Delay1/1, Relational Operator2/1
  Relational Operator2/1 -> Switch/2
  uint2/1 -> MinMax/2
  Unit Delay1/1 -> Relational Operator2/2
  uint32/1 -> Switch/1
  Unit Delay2/1 -> Sum1/2
  product/1 -> Relational Operator/1, HvCoorn_tiHVPStTimer/1  "HvCoorn_tiHVPStTimer"
  uint1/1 -> Sum1/1
  Switch/1 -> Unit Delay2/1, DataTypeConversion/1
  MinMax/1 -> Switch/3
  Sum1/1 -> MinMax/1
  DataTypeConversion/1 -> product/1
  AND/1 -> OR/1
  OR/1 -> Logical Operator/3
  sup_tiWaitIgnOn_C1/1 -> OR/2
  OR1/1 -> Logical Operator/4
  HvCoorn_bHvRlyOpenAct/1 -> OR1/1
  sup_tiWaitIgnOn_C2/1 -> OR1/2

== system HvCoorn/HvCoorn/HVP_HighVoltagePowerOnOffProcedure/A03_Comm2HVReqCal ==
  note: Documentation
  PwrLimBatt_pwrMaxHvesDChrg : Inport
  ian_uSupBattVolt : Inport  Port=2
  icbms_bPrecResOverTemp : Inport  Port=3
  icbms_pctHVBatSOCDisp : Inport  Port=4
  GearLvr_stDrvGear : Inport  Port=5
  icbms_stHvBat : Inport  Port=6
  icdc_stMode : Inport  Port=7
  icfm_stMode : Inport  Port=8
  icobc_stOBCMode : Inport  Port=9
  HvCoorn_tiHVPStTimer : Inport  Port=10
  HvCoorn_bHvilStOk : Inport  Port=11
  HvCoorn_bStartUpReq : Inport  Port=12
  HvCoorn_bObcChrgrCnct : Inport  Port=13
  HvCoorn_stHVPOld : Inport  Port=14
  idi_bKeyOn : Inport  Port=15
  HvCoorn_bDCChrgLink : Inport  Port=16
  icrm_stMode : Inport  Port=17
  ipf_bPCAN0x130Vld : Inport  Port=18
  ipf_bPCAN0x111S1Vld : Inport  Port=19
  DTC_bDiagEnaCdnWkupSho : Inport  Port=20
  DTC_bDiagRst : Inport  Port=21
  HvCoorn_bHvOnFailRst : Inport  Port=22
  AND1 : Logic  Inputs=4  OutDataTypeStr=boolean
  AND2 : Logic  Operator=OR  Inputs=3  OutDataTypeStr=boolean
  AND4 : Logic  Operator=NOT  OutDataTypeStr=boolean
  Calibration1 : Constant  Description=[0]  Value=HvCoorn_bHvInitFailEna_C  SampleTime=-1
      settings: AttributesFormatString=%<Description>
  Calibration6 : Constant  Description=[9999]  Value=HvCoorn_rHvInitFailThd_C  SampleTime=-1
      settings: AttributesFormatString=%<Description>
  Calibration7 : Constant  Description=[1]  Value=HvCoorn_rHvInitRcv_C  SampleTime=-1
      settings: AttributesFormatString=%<Description>
  Copyright : simulink/Model-Wide Utilities/Model Info  Frame=on  DisplayStringWithTags=|  HorizontalTextAlignment=Left  LeftAlignmentValue=0.02
      | © ITK Engineering Technology (Wu Xi) Co., Ltd. (ITKC)
      | 
      | Model Version: %<ModelVersion>
      | Date: %<LastModificationDate>
  DebCnt : ITKLib/TimeCounter/DebCnt
      settings: SourceProductName=ITKC_Lib
  HysteresisA : ITKLib/Hysteresis/HysteresisA  Description=HysteresisA
      settings: AttributesFormatString=%<Description>  SourceProductName=ITKC_Lib
  InlineDescription : ITKLib/Special/InlineDescription  Tag=HideFromReport  Description=通讯连接跳转至高压请求  ShowInLibBrowser=0  RefreshPar=0
      settings: SourceProductName=ITKC_Lib
  Logical Operator{1,4,17,19,24} (5 alike) : Logic  Operator=NOT  Inputs=1  AllPortsSameDT=off  OutDataTypeStr=boolean
  Logical Operator{8..10,12..14,16,18,20..21} (10 alike) : Logic  Operator=OR  AllPortsSameDT=off  OutDataTypeStr=boolean
  Logical Operator{5,11,15,23} (4 alike) : Logic  AllPortsSameDT=off  OutDataTypeStr=boolean
  Logical Operator2 : Logic  Inputs=3  AllPortsSameDT=off  OutDataTypeStr=boolean
  Logical Operator3 : Logic  Operator=OR  Inputs=3  AllPortsSameDT=off  OutDataTypeStr=boolean
  Logical Operator6 : Logic  Inputs=6  AllPortsSameDT=off  OutDataTypeStr=boolean
  Logical Operator7 : Logic  Inputs=4  AllPortsSameDT=off  OutDataTypeStr=boolean
  Lower : RelationalOperator  Operator=<  OutDataTypeStr=boolean
  RSLatch : ITKLib/Memory/RSLatch
      settings: SourceProductName=ITKC_Lib
  Relational Operator{1..3,5,7,11..16,18..19} (13 alike) : RelationalOperator  Operator===  OutDataTypeStr=boolean  InputSameDT=off
  Relational Operator10 : RelationalOperator  Operator=>  OutDataTypeStr=boolean  InputSameDT=off
  Relational Operator17 : RelationalOperator  Operator=>  OutDataTypeStr=boolean  InputSameDT=off
  Relational Operator4 : RelationalOperator  OutDataTypeStr=boolean  InputSameDT=off
  Subtract1 : Sum  Inputs=+-  InputSameDT=on  SaturateOnIntegerOverflow=on
  Switch1 : Switch  Criteria=u2 ~= 0  SaturateOnIntegerOverflow=off  InputSameDT=off
  Switch2 : Switch  Criteria=u2 ~= 0  SaturateOnIntegerOverflow=off  InputSameDT=off
  Switch3 : Switch  Criteria=u2 ~= 0  SaturateOnIntegerOverflow=off  InputSameDT=off
  TRUE : Constant  Description=TRUE  OutDataTypeStr=boolean
      settings: AttributesFormatString=%<Description>
  TRUE1 : Constant  Description=TRUE  OutDataTypeStr=boolean
      settings: AttributesFormatString=%<Description>
  TRUE2 : Constant  Description=TRUE  OutDataTypeStr=boolean
      settings: AttributesFormatString=%<Description>
  TaskTime_s1 : Constant  Value=TaskTime_10ms
      settings: AttributesFormatString=[0.01]
  TurnOnDelayVari : ITKLib/TimeCounter/TurnOnDelayVari
      settings: AttributesFormatString=TurnOnDelay  SourceProductName=ITKC_Lib
  Unit detailed design : simulink/Model-Wide Utilities/DocBlock  Tag=HideFromReport  DocumentType=Text
      content=|
      | SMiVCU-3282 - 通讯连接跳转至高压请求标志位
      | 以下条件同时满足，则激活[通讯连接跳转至高压请求标志位]：
      | 1.<电池状态>为0x1：Off Line或0x6：Disconnect；
      | 2.<DCDC状态>为0x1：Disconnect或0x2：Connected；
      | 3.<前电机状态>为0x1：Initial或0x2：Standby（两驱时屏蔽）；
      | 4.<后电机状态>为0x1：Initial或0x2：Standby；
      | 5.[状态持续时间]大于一定值（HvCoorn_tiWait4Comm_C，初始值0.02s）；
      | 6.[高压互锁OK标志位]为1；
      | 7.<OBC充电连接状态>为0x2：Connected、0x3：V2VConnected、0x4：V2LConnected时，<OBC状态>为0x1：Disconnect或0x2：Connected；
      | 8.<OBC充电连接状态>不为0x2：Connected、0x3：V2VConnected、0x4：V2LConnected且[DC充电连接标志位]为0时，<电池SOC>大于一定值（HvCoorn_pctSocAdj4HvOn_C，初始值-1)且<电池最大放电功率>大于一定值（HvCoorn_pwrBatDChrg4HvOn_C，初始值-1000W）；
      | 9.<整车电源模式>为0x1：On时<VCU内部实际挡位状态>为0x4：N或0x6：P；
      |
      | SMiVCU-3284 - 高压初始化失败标志位
      | [通讯连接跳转至高压请求标志位]为0且上一时刻<高压系统状态>为0x11：Wait4Communication，TurnOnDelay一定时间（HvCoorn_tiHvInitFailSet_C，5s）后激活并锁存[高压初始化失败标志位]，待[上高压需求标志位]出现上升沿后Reset。
      |
      | SMiVCU-3288 - 通讯跳转至关闭ECU标志位
      | [高压初始化失败标志位]为1，或[上高压需求标志位]为0，则激活[通讯跳转至关闭ECU标志位]。
  icbms_offline : Constant  Description=[1]  Value=BMSActSt_offline
      settings: AttributesFormatString=[1]
  icbms_offline1 : Constant  Description=[6]  Value=BMSActSt_disconnect
      settings: AttributesFormatString=[6]
  icdc_connected : Constant  Description=[2]  Value=DCDCActSt_connected
      settings: AttributesFormatString=[2]
  icdc_disconnected : Constant  Description=[1]  Value=DCDCActSt_disconnected
      settings: AttributesFormatString=[1]
  icm_standby : Constant  Description=[2]  Value=MCUActSt_standby
      settings: AttributesFormatString=[2]
  icm_standby1 : Constant  Description=[2]  Value=MCUActSt_standby
      settings: AttributesFormatString=[2]
  icm_standby2 : Constant  Description=[1]  Value=MCUActSt_init
      settings: AttributesFormatString=[1]
  icm_standby3 : Constant  Description=[1]  Value=MCUActSt_init
      settings: AttributesFormatString=[1]
  icobc_connected : Constant  Description=[2]  Value=OBCActSt_connected
      settings: AttributesFormatString=[2]
  icobc_disconnected : Constant  Description=[1]  Value=OBCActSt_disconnected
      settings: AttributesFormatString=[1]
  int1 : Constant  Value=-1  OutDataTypeStr=int16  SampleTime=-1
      settings: AttributesFormatString=%<OutDataTypeStr>
  int16 : Constant  OutDataTypeStr=int16  SampleTime=-1
      settings: AttributesFormatString=%<OutDataTypeStr>
  sup_bHVReqEnaMan_C : Constant  Description=[1]  Value=HvCoorn_bHVReqEnaMan_C  OutDataTypeStr=boolean
      settings: AttributesFormatString=%<Description>
  sup_bHVReqGearDisable_C : Constant  Description=[0]  Value=HvCoorn_bHVReqGearDisable_C
      settings: AttributesFormatString=%<Description>
  sup_percSocAdj4HvOn_C : Constant  Description=[-1]  Value=HvCoorn_pctSocAdj4HvOn_C
      settings: AttributesFormatString=%<Description>
  sup_pwrBatDchg4HvOn_C : Constant  Description=[-1000]  Value=HvCoorn_pwrBatDChrg4HvOn_C
      settings: AttributesFormatString=%<Description>
  sup_pwrBatDchg4HvOn_C1 : Constant  Description=[6]  Value=GearLvr_stDrvGearP_SC
      settings: AttributesFormatString=%<Description>
  sup_pwrBatDchg4HvOn_C2 : Constant  Description=[4]  Value=GearLvr_stDrvGearN_SC
      settings: AttributesFormatString=%<Description>
  sup_tiWait4Comm_C : Constant  Description=[0.02]  Value=HvCoorn_tiWait4Comm_C
      settings: AttributesFormatString=%<Description>
  sup_tiWaitPrecResTemp_C : Constant  Description=[3]  Value=HvCoorn_tiWaitPrecResTemp_C
      settings: AttributesFormatString=%<Description>
  sup_vLowBatVoltLim_C : Constant  Description=[6]  Value=HvCoorn_uLoThdLvBatVolt_C
      settings: AttributesFormatString=%<Description>
  sup_vLowBatVoltLim_C1 : Constant  Description=[9]  Value=HvCoorn_uHiThdLvBatVolt_C
      settings: AttributesFormatString=%<Description>
  sup_vLowBatVoltLim_C2 : Constant  Description=[16]  Value=HvCoorn_uMaxLvBatVolt_C
      settings: AttributesFormatString=%<Description>
  sup_vLowBatVoltLim_C3 : Constant  Description=[1]  Value=HvCoorn_bHvOnDCDCByp_C
      settings: AttributesFormatString=%<Description>
  uint3 : Constant  Description=Wait4Communication  Value=11  OutDataTypeStr=uint8
      settings: AttributesFormatString=|
      | %<OutDataTypeStr>
      | %<Description>
  HvCoorn_bHvInitFail : Outport  VectorParamsAs1DForOutWhenUnconnected=off
  HvCoorn_bComm2HVReq : Outport  Port=2  VectorParamsAs1DForOutWhenUnconnected=off
  HvCoorn_bComm2ShutECU : Outport  Port=3  VectorParamsAs1DForOutWhenUnconnected=off
  wires:
  icbms_stHvBat/1 -> Relational Operator18/1, Relational Operator1/1
  Relational Operator1/1 -> Logical Operator21/1
  HvCoorn_tiHVPStTimer/1 -> Relational Operator4/1
  sup_tiWait4Comm_C/1 -> Relational Operator4/2
  icdc_disconnected/1 -> Relational Operator5/2
  Relational Operator4/1 -> Logical Operator7/3
  HvCoorn_bHvilStOk/1 -> Logical Operator7/4
  icfm_stMode/1 -> Relational Operator3/1, Relational Operator7/1
  icm_standby/1 -> Relational Operator7/2
  Relational Operator7/1 -> Logical Operator8/1
  sup_vLowBatVoltLim_C/1 -> HysteresisA/3
  HysteresisA/1 -> Logical Operator7/1
  ian_uSupBattVolt/1 -> Lower/1, HysteresisA/2
  sup_tiWaitPrecResTemp_C/1 -> TurnOnDelayVari/3
  icbms_bPrecResOverTemp/1 -> Logical Operator15/1, Logical Operator4/1
  Logical Operator4/1 -> Logical Operator5/1  "bPrecResOverTempOK"
  Logical Operator7/1 -> Logical Operator6/2  "bVehOk"
  Logical Operator5/1 -> Logical Operator6/6  "bPrecResOk"
  Logical Operator2/1 -> Logical Operator6/1  "bHvCompOk"
  sup_bHVReqEnaMan_C/1 -> Logical Operator9/2
  Logical Operator9/1 -> HvCoorn_bComm2HVReq/1  "HvCoorn_bComm2HVReq"
  TurnOnDelayVari/1 -> RSLatch/1
  Logical Operator24/1 -> Logical Operator5/2
  icbms_pctHVBatSOCDisp/1 -> Relational Operator10/1
  Switch2/1 -> Logical Operator6/4  "bSocOk"
  icobc_disconnected/1 -> Relational Operator11/2
  icobc_stOBCMode/1 -> Relational Operator11/1, Relational Operator12/1
  icobc_connected/1 -> Relational Operator12/2
  Relational Operator11/1 -> Logical Operator12/1
  Relational Operator12/1 -> Logical Operator12/2
  Logical Operator12/1 -> Switch3/1
  Switch3/1 -> Logical Operator6/3  "bObcOk"
  GearLvr_stDrvGear/1 -> Relational Operator13/1, Relational Operator14/1
  sup_pwrBatDchg4HvOn_C1/1 -> Relational Operator13/2
  sup_pwrBatDchg4HvOn_C2/1 -> Relational Operator14/2
  Relational Operator13/1 -> Logical Operator14/1
  Relational Operator14/1 -> Logical Operator14/2
  Logical Operator13/1 -> Logical Operator6/5  "bGearOk"
  HvCoorn_stHVPOld/1 -> Relational Operator15/1
  uint3/1 -> Relational Operator15/2
  icdc_connected/1 -> Relational Operator16/2
  Relational Operator5/1 -> Logical Operator3/1
  Relational Operator16/1 -> Logical Operator3/2
  Logical Operator3/1 -> Logical Operator2/2
  TRUE/1 -> Switch3/3
  sup_bHVReqGearDisable_C/1 -> Logical Operator13/2
  idi_bKeyOn/1 -> Switch1/2
  TRUE2/1 -> Switch1/3
  Switch1/1 -> Logical Operator13/1
  Logical Operator14/1 -> Switch1/1
  HvCoorn_bObcChrgrCnct/1 -> Switch3/2, Logical Operator10/1
  Logical Operator1/1 -> Switch2/2
  Logical Operator23/1 -> Switch2/1
  TRUE1/1 -> Switch2/3
  HvCoorn_bStartUpReq/1 -> Logical Operator19/1
  Logical Operator6/1 -> Logical Operator17/1, Logical Operator9/1
  Relational Operator15/1 -> Logical Operator15/2, Logical Operator11/2
  HvCoorn_bHvOnFailRst/1 -> RSLatch/2, AND2/2
  Logical Operator17/1 -> Logical Operator11/1
  Logical Operator19/1 -> Logical Operator18/2
  Logical Operator18/1 -> HvCoorn_bComm2ShutECU/1  "HvCoorn_bComm2ShutECU"
  sup_percSocAdj4HvOn_C/1 -> Relational Operator10/2
  RSLatch/1 -> Logical Operator24/1
  icdc_stMode/1 -> Relational Operator5/1, Relational Operator16/1
  PwrLimBatt_pwrMaxHvesDChrg/1 -> Relational Operator17/1
  sup_pwrBatDchg4HvOn_C/1 -> Relational Operator17/2
  Relational Operator10/1 -> Logical Operator23/1
  Relational Operator17/1 -> Logical Operator23/2
  icbms_offline/1 -> Relational Operator1/2
  HvCoorn_bDCChrgLink/1 -> Logical Operator10/2
  Logical Operator10/1 -> Logical Operator1/1
  TaskTime_s1/1 -> TurnOnDelayVari/2
  Logical Operator15/1 -> TurnOnDelayVari/1
  icm_standby1/1 -> Relational Operator19/2
  icrm_stMode/1 -> Relational Operator2/1, Relational Operator19/1
  Logical Operator20/1 -> Logical Operator16/2
  Logical Operator16/1 -> Logical Operator2/3
  Relational Operator19/1 -> Logical Operator20/1
  icm_standby2/1 -> Relational Operator2/2
  Relational Operator2/1 -> Logical Operator20/2
  icm_standby3/1 -> Relational Operator3/2
  Relational Operator3/1 -> Logical Operator8/2
  Logical Operator21/1 -> Logical Operator2/1
  icbms_offline1/1 -> Relational Operator18/2
  Relational Operator18/1 -> Logical Operator21/2
  sup_vLowBatVoltLim_C1/1 -> HysteresisA/1
  Lower/1 -> Logical Operator7/2
  sup_vLowBatVoltLim_C2/1 -> Lower/2
  ipf_bPCAN0x111S1Vld/1 -> AND1/3
  ipf_bPCAN0x130Vld/1 -> AND1/2
  DTC_bDiagEnaCdnWkupSho/1 -> AND1/1
  Logical Operator8/1 -> Logical Operator16/1
  sup_vLowBatVoltLim_C3/1 -> Logical Operator3/3
  Calibration7/1 -> Subtract1/2
  Subtract1/1 -> DebCnt/5
  DebCnt/1 -> HvCoorn_bHvInitFail/1, Logical Operator18/1
  AND2/1 -> DebCnt/2
  int16/1 -> DebCnt/6
  AND4/1 -> AND2/3
  DTC_bDiagRst/1 -> AND2/1
  Logical Operator11/1 -> DebCnt/1
  AND1/1 -> AND4/1, DebCnt/3
  int1/1 -> DebCnt/7
  Calibration6/1 -> Subtract1/1, DebCnt/4
  Calibration1/1 -> AND1/4
